simulink model "Ejemplo9_17"  (R2021b)
settings: Solver=ode4  StartTime=0.0  StopTime=20  FixedStep=0.01  RelTol=1e-3
settings Model: Creator=cesar  LastModifiedBy=cesar

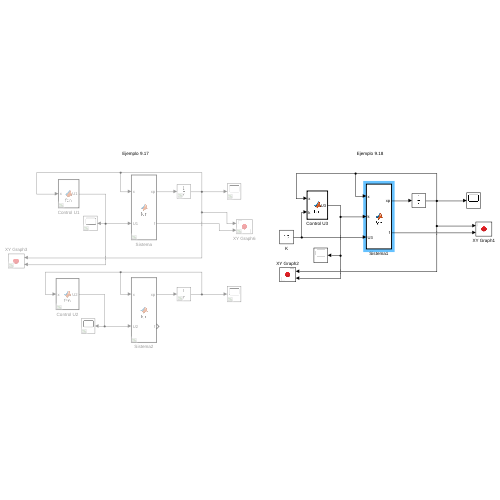
[thumbnail: Simulink's stored preview of the top-level diagram]
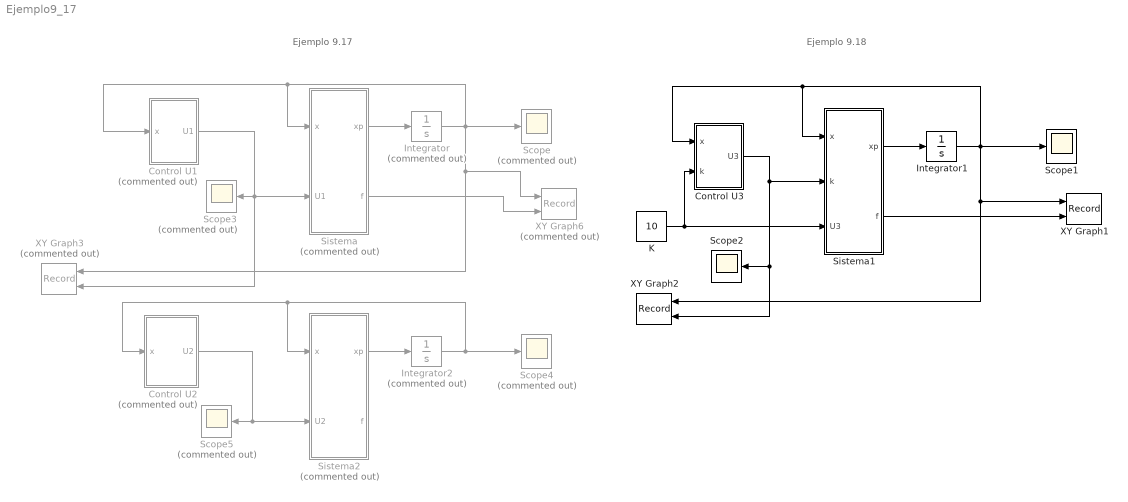
== system Ejemplo9_17 ==
  note: Ejemplo 9.17
  note: Ejemplo 9.18
  Control U1 : MATLAB Function  Commented=on  TreatAsAtomicUnit=on
  Control U2 : MATLAB Function  Commented=on  TreatAsAtomicUnit=on
  Control U3 : MATLAB Function  TreatAsAtomicUnit=on
  Integrator : Integrator  Commented=on
  Integrator1 : Integrator  InitialCondition=5
  Integrator2 : Integrator  Commented=on
  K : Constant  Value=10
  Scope{,3..5} (4 alike) : Scope  Commented=on
  Scope1 : Scope
  Scope2 : Scope
  Sistema : MATLAB Function  Commented=on  TreatAsAtomicUnit=on
  Sistema1 : MATLAB Function  TreatAsAtomicUnit=on
  Sistema2 : MATLAB Function  Commented=on  TreatAsAtomicUnit=on
  XY Graph1 : Record  FileSettingsInternal="{\"entries\":[{\"content\":{\"excelSettings\":{\"content\":{},\"type\":\"Streamout.ExcelSettings\"}},\"type\":\"Streamout.FileSettingStorage\",\"uuid\":\"285d6b9e-57d1-4632-8a93-13e0081877e7\"}],\"packageUris\":[\"http://schema.mathworks.com/mf0/streamout_blocks/R2020a\"],\"version\":\"1.0\"}"  Layout=[1 1]  SignalsInternal="{\"entries\":[{\"content\":{\"signals\":[{\"content\":{\"blockPath\":[\"Ejemplo9_17/XY Graph1\"],\"channel\":[],\"dimensions\":[1],\"domain\":\"Ejemplo9_17/XY Graph1\",\"lineColor\":\"#a2142f\",\"plots\":[1],\"port\":1,\"sid\":[\"\"],\"signalID\":1705,\"signalName\":\"Integrator1\"},\"type\":\"RecordBlkView.Signal\",\"uuid\":\"b971d81f-d9f7-40d6-91f8-4ea20e89d19d\"},{\"content\":{\"blockPath\":[\"Ejemplo9_17/XY Graph1\"],\"channel\":[],\"dimensions\":[1],\"domain\":\"Ejemplo9_17/XY Graph1\",\"lineColor\":\"#139fff\",\"plots\":[1],\"port\":2,\"sid\":[\"\"],\"signalID\":1709,\"signalName\":\"Sistema1:2\"},\"type\":\"RecordBlkView.Signal\",\"uuid\":\"6aa58497-6415-41a1-a392-6edf0e9941e6\"}]},\"type\":\"RecordBlkView.InputSignals\",\"uuid\":\"496dce93-78b1-4470-8a6c-bab7a5205eac\"}],\"packageUris\":[\"http://schema.mathworks.com/mf0/streamout_blocks/R2020a\"],\"version\":\"1.0\"}"  VisualizationBindings="{\"xyplotplugin\":{\"info\":[{\"series\":[{\"bindingParametersList\":[{\"parameter\":\"X-Axis\",\"signalID\":1705,\"signalName\":\"Integrator1\"},{\"parameter\":\"Y-Axis\",\"signalID\":1709,\"signalName\":\"Sistema1:2\"}],\"seriesID\":64494}],\"subplotID\":1}]}}"  CompatibilityTag=XY
  XY Graph2 : Record  FileSettingsInternal="{\"entries\":[{\"content\":{\"excelSettings\":{\"content\":{},\"type\":\"Streamout.ExcelSettings\"}},\"type\":\"Streamout.FileSettingStorage\",\"uuid\":\"26f140e9-1351-4ae6-b296-d34ac1091e77\"}],\"packageUris\":[\"http://schema.mathworks.com/mf0/streamout_blocks/R2020a\"],\"version\":\"1.0\"}"  Layout=[1 1]  SignalsInternal="{\"entries\":[{\"content\":{\"signals\":[{\"content\":{\"blockPath\":[\"Ejemplo9_17/XY Graph2\"],\"channel\":[],\"dimensions\":[1],\"domain\":\"Ejemplo9_17/XY Graph2\",\"lineColor\":\"#a2142f\",\"plots\":[1],\"port\":1,\"sid\":[\"\"],\"signalID\":1713,\"signalName\":\"Integrator1\"},\"type\":\"RecordBlkView.Signal\",\"uuid\":\"a629b91d-a06a-49b2-8b15-1d3397dd949a\"},{\"content\":{\"blockPath\":[\"Ejemplo9_17/XY Graph2\"],\"channel\":[],\"dimensions\":[1],\"domain\":\"Ejemplo9_17/XY Graph2\",\"lineColor\":\"#139fff\",\"plots\":[1],\"port\":2,\"sid\":[\"\"],\"signalID\":1717,\"signalName\":\"Control U3\"},\"type\":\"RecordBlkView.Signal\",\"uuid\":\"f97fd613-a85c-44d9-8b17-e6845e80be1d\"}]},\"type\":\"RecordBlkView.InputSignals\",\"uuid\":\"9c024509-0a66-40bc-8c8c-d67ab64a8a43\"}],\"packageUris\":[\"http://schema.mathworks.com/mf0/streamout_blocks/R2020a\"],\"version\":\"1.0\"}"  VisualizationBindings="{\"xyplotplugin\":{\"info\":[{\"series\":[{\"bindingParametersList\":[{\"parameter\":\"X-Axis\",\"signalID\":1713,\"signalName\":\"Integrator1\"},{\"parameter\":\"Y-Axis\",\"signalID\":1717,\"signalName\":\"Control U3\"}],\"seriesID\":57647}],\"subplotID\":1}]}}"  CompatibilityTag=XY
  XY Graph3 : Record  Commented=on  FileSettingsInternal="{\"entries\":[{\"content\":{\"excelSettings\":{\"content\":{},\"type\":\"Streamout.ExcelSettings\"}},\"type\":\"Streamout.FileSettingStorage\",\"uuid\":\"9eca84eb-f65d-48ee-b887-62351bee95d2\"}],\"packageUris\":[\"http://schema.mathworks.com/mf0/streamout_blocks/R2020a\"],\"version\":\"1.0\"}"  Layout=[1 1]  SignalsInternal="{\"entries\":[{\"content\":{\"signals\":[]},\"type\":\"RecordBlkView.InputSignals\",\"uuid\":\"570572f3-645f-4ac6-a4b6-cb3f22f652ff\"}],\"packageUris\":[\"http://schema.mathworks.com/mf0/streamout_blocks/R2020a\"],\"version\":\"1.0\"}"  VisualizationBindings="{\"xyplotplugin\":{\"info\":[{\"series\":[],\"subplotID\":1}]}}"  CompatibilityTag=XY
  XY Graph6 : Record  Commented=on  FileSettingsInternal="{\"entries\":[{\"content\":{\"excelSettings\":{\"content\":{},\"type\":\"Streamout.ExcelSettings\"}},\"type\":\"Streamout.FileSettingStorage\",\"uuid\":\"ba308264-28e2-4c27-9ec6-c68c1152fc21\"}],\"packageUris\":[\"http://schema.mathworks.com/mf0/streamout_blocks/R2020a\"],\"version\":\"1.0\"}"  Layout=[1 1]  SignalsInternal="{\"entries\":[{\"content\":{\"signals\":[]},\"type\":\"RecordBlkView.InputSignals\",\"uuid\":\"f3679a38-62a2-4b76-8e8f-39a71b715a56\"}],\"packageUris\":[\"http://schema.mathworks.com/mf0/streamout_blocks/R2020a\"],\"version\":\"1.0\"}"  VisualizationBindings="{\"xyplotplugin\":{\"info\":[{\"series\":[],\"subplotID\":1}]}}"  CompatibilityTag=XY
  wires:
  Control U1/1(U1) -> XY Graph3/2, Sistema/2(U1), Scope3/1
  Sistema/1(xp) -> Integrator/1
  Integrator/1 -> XY Graph6/1, XY Graph3/1, Sistema/1(x), Control U1/1(x), Scope/1
  Sistema1/1(xp) -> Integrator1/1
  Control U3/1(U3) -> XY Graph2/2, Scope2/1, Sistema1/2(k)
  Integrator1/1 -> Scope1/1, XY Graph2/1, XY Graph1/1, Sistema1/1(x), Control U3/1(x)
  K/1 -> Control U3/2(k), Sistema1/3(U3)
  Control U2/1(U2) -> Sistema2/2(U2), Scope5/1
  Sistema2/1(xp) -> Integrator2/1
  Integrator2/1 -> Scope4/1, Control U2/1(x), Sistema2/1(x)
  Sistema1/2(f) -> XY Graph1/2
  Sistema/2(f) -> XY Graph6/2

== matlab function Ejemplo9_17/Sistema ==
  data: x input; xp output; U1 input; f output
function [xp,f]  = fcn(x,U1)

xp = x - x^3 + U1;
f = x - x^3;
end

== matlab function Ejemplo9_17/Control U2 ==
  data: U2 output; x input
function U2    = fcn(x)

U2 = -x + (x)^3 - x*sqrt( (1-(x)^2)^2 +1);

== matlab function Ejemplo9_17/Control U1 ==
  data: U1 output; x input
function U1   = fcn(x)

alpha = sqrt(2);
U1 = -x + (x)^3 -alpha*x;
end

== matlab function Ejemplo9_17/Control U3 ==
  data: U3 output; x input; k input
function U3   = fcn(x,k) 
alpha = sqrt(2);
U3 = (1/k)*(-x + (x)^3 -alpha*k*x -k*x + x);
end

== matlab function Ejemplo9_17/Sistema1 ==
  data: x input; xp output; k input; U3 input; f output
function [xp,f]  = fcn(x,k,U3)

xp = x - x^3 + sin(x)*k*U3;
f = x - x^3;
end

== matlab function Ejemplo9_17/Sistema2 ==
  data: x input; xp output; U2 input; f output
function [xp,f]  = fcn(x,U2)

xp = x - x^3 + U2;
%xp = x - x^3 + U2;
f = x - x^3;
end
